simulink model "SC_617_HOMEWORK_2"  (R2025a)
settings: Solver=VariableStepAuto  StartTime=0.0  StopTime=50  RelTol=1e-3
InitFcn:
  | init_params
values from neighbouring files (symbols this model uses):
  A1 = 0.4 * I3    [init_params.m]
  A2 = 0.1 * I3    [init_params.m]
  G = [0; 0; -g]    [init_params.m]
  J = diag([0.00235, 0.00235, 0.0526])    [init_params.m]
  J_inv = inv(J)    [init_params.m]
  K1 = 1 * I3    [init_params.m]
  K2 = 0.01 * I3    [init_params.m]
  X1 = -A1*A1 + I3    [init_params.m]
  X2 = -A2*A2 + I3    [init_params.m]
  Y1 = A1 + Q1 + K1    [init_params.m]
  Y2 = A2 + Q2 + K2    [init_params.m]
libraries: matrix_library x1
settings Model: Creator=bhuvn  LastModifiedBy=bhuvn

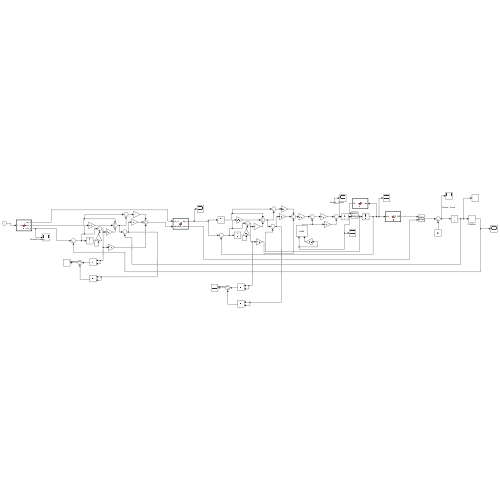
[thumbnail: Simulink's stored preview of the top-level diagram]
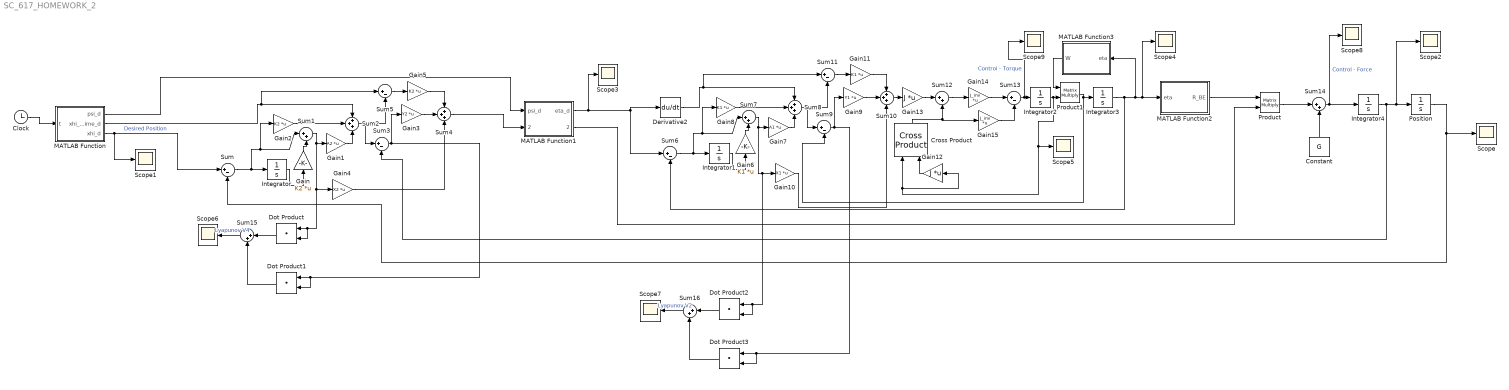
== system SC_617_HOMEWORK_2 ==
  Clock : Clock
  Constant : Constant  Value=G
  Cross Product : matrix_library/Cross Product
  Derivative2 : Derivative
  Dot Product{,1..3} (4 alike) : DotProduct  OutDataTypeStr=Inherit: Inherit via internal rule
  Gain : Gain  Gain=K2  Multiplication=Matrix(K*u)
  Gain1 : Gain  Gain=A2  Multiplication=Matrix(K*u)
  Gain10 : Gain  Gain=X1  Multiplication=Matrix(K*u)
  Gain11 : Gain  Gain=K1  Multiplication=Matrix(K*u)
  Gain12 : Gain  Gain=J  Multiplication=Matrix(K*u)
  Gain13 : Gain  Gain=J  Multiplication=Matrix(K*u)
  Gain14 : Gain  Gain=J_inv  Multiplication=Matrix(K*u)
  Gain15 : Gain  Gain=J_inv  Multiplication=Matrix(K*u)
  Gain2 : Gain  Gain=K2  Multiplication=Matrix(K*u)
  Gain3 : Gain  Gain=Y2  Multiplication=Matrix(K*u)
  Gain4 : Gain  Gain=X2  Multiplication=Matrix(K*u)
  Gain5 : Gain  Gain=K2  Multiplication=Matrix(K*u)
  Gain6 : Gain  Gain=K1  Multiplication=Matrix(K*u)
  Gain7 : Gain  Gain=A1  Multiplication=Matrix(K*u)
  Gain8 : Gain  Gain=K1  Multiplication=Matrix(K*u)
  Gain9 : Gain  Gain=Y1  Multiplication=Matrix(K*u)
  Integrator{,1..4} (5 alike) : Integrator
  MATLAB Function : MATLAB Function  TreatAsAtomicUnit=on
  MATLAB Function1 : MATLAB Function  TreatAsAtomicUnit=on
  MATLAB Function2 : MATLAB Function  TreatAsAtomicUnit=on
  MATLAB Function3 : MATLAB Function  TreatAsAtomicUnit=on
  Position : Integrator  ContinuousStateAttributes="\"\""
  Product : Product  Multiplication=Matrix(*)
  Product1 : Product  Multiplication=Matrix(*)
  Scope{,1..9} (10 alike) : Scope
      Scope settings: ActiveDisplayYMinimum=-4.4635582145538866  ActiveDisplayYMaximum=9.864933478588199
      Scope1 settings: ActiveDisplayYMinimum=-8.7534376610536011  ActiveDisplayYMaximum=9.9256887521870869
      Scope2 settings: ActiveDisplayYMinimum=-1.1742628607223897  ActiveDisplayYMaximum=2.1905461290166537  DataLoggingVariableName=ScopeData2
      Scope3 settings: ActiveDisplayYMinimum=-0.36738889438246891  ActiveDisplayYMaximum=0.46299980810775304  DataLoggingVariableName=ScopeData3
      Scope4 settings: ActiveDisplayYMinimum=-0.8680947606325895  ActiveDisplayYMaximum=0.33111411374778932  DataLoggingVariableName=ScopeData4
      Scope5 settings: ActiveDisplayYMinimum=-5.3845863313289479  ActiveDisplayYMaximum=8.3533958672384383  DataLoggingVariableName=ScopeData5
      Scope6 settings: ActiveDisplayYMinimum=0.017644834477093529  ActiveDisplayYMaximum=1.7083666755814968  DataLoggingVariableName=ScopeData6
      Scope7 settings: ActiveDisplayYMinimum=-0.096269739376810465  ActiveDisplayYMaximum=0.17835060014207538  DataLoggingVariableName=ScopeData7
      Scope8 settings: ActiveDisplayYMinimum=-1.5602667584024623  ActiveDisplayYMaximum=1.6746897222216022  DataLoggingVariableName=ScopeData8
      Scope9 settings: ActiveDisplayYMinimum=-0.8680947606325895  ActiveDisplayYMaximum=0.33111411374778932  DataLoggingVariableName=ScopeData9
  Sum{,3,5..6,9,11,13} (7 alike) : Sum  Inputs=|+-
  Sum{1,7,12,14..16} (6 alike) : Sum  Inputs=|++
  Sum{2,4,8,10} (4 alike) : Sum  Inputs=+++
  wires:
  Clock/1 -> MATLAB Function/1(t)
  MATLAB Function/3(xhi_d) -> Scope1/1, Sum/1  "Desired Position"
  Sum/1 -> Sum1/1, Gain2/1, Integrator/1
  Gain/1 -> Sum1/2
  Integrator/1 -> Gain/1
  MATLAB Function/2(xhi_prime_d) -> Sum5/1, Sum2/1
  Sum1/1 -> Dot Product/2, Dot Product/1, Gain4/1, Gain1/1
  Gain1/1 -> Sum2/3
  Gain2/1 -> Sum2/2
  Sum2/1 -> Sum5/2, Sum3/1
  Sum3/1 -> Gain3/1, Dot Product1/2, Dot Product1/1
  Gain3/1 -> Sum4/2
  Gain4/1 -> Sum4/3
  Sum5/1 -> Gain5/1
  Gain5/1 -> Sum4/1
  MATLAB Function/1(psi_d) -> MATLAB Function1/1(psi_d)
  Gain10/1 -> Sum10/3
  Sum11/1 -> Gain11/1
  Gain11/1 -> Sum10/1
  Integrator1/1 -> Gain6/1
  Gain7/1 -> Sum8/3
  Derivative2/1 -> Sum11/1, Sum8/1
  Gain8/1 -> Sum8/2
  Sum6/1 -> Sum7/1, Gain8/1, Integrator1/1
  Gain9/1 -> Sum10/2
  Sum9/1 -> Dot Product3/2, Dot Product3/1, Gain9/1
  Sum8/1 -> Sum11/2, Sum9/1
  Gain6/1 -> Sum7/2
  Sum7/1 -> Dot Product2/2, Dot Product2/1, Gain10/1, Gain7/1
  Cross Product/1 -> Gain15/1, Sum12/2
  Sum10/1 -> Gain13/1
  Gain13/1 -> Sum12/1
  Sum12/1 -> Gain14/1
  Gain14/1 -> Sum13/1
  Sum13/1 -> Scope9/1, Integrator2/1  "Control - Torque"
  Integrator3/1 -> Sum6/2, MATLAB Function3/1(eta), MATLAB Function2/1(eta), Scope4/1
  MATLAB Function2/1(R_BE) -> Product/1
  Product/1 -> Sum14/1
  Sum14/1 -> Integrator4/1, Scope8/1  "Control - Force"
  Integrator4/1 -> Sum3/2, Scope2/1, Position/1
  Position/1 -> Sum/2, Scope/1
  Integrator2/1 -> Scope5/1, Cross Product/1, Gain12/1, Product1/2
  Product1/1 -> Sum9/2, Integrator3/1
  MATLAB Function3/1(W) -> Product1/1
  MATLAB Function1/1(eta_d) -> Scope3/1, Sum6/1, Derivative2/1
  MATLAB Function1/2(L_vector) -> Product/2
  Gain15/1 -> Sum13/2
  Gain12/1 -> Cross Product/2
  Constant/1 -> Sum14/2
  Sum4/1 -> MATLAB Function1/2(alpha4)
  Dot Product/1 -> Sum15/1
  Dot Product1/1 -> Sum15/2
  Sum15/1 -> Scope6/1  "Lyapunov V4"
  Sum16/1 -> Scope7/1  "Lyapunov V2"
  Dot Product2/1 -> Sum16/1
  Dot Product3/1 -> Sum16/2

== matlab function SC_617_HOMEWORK_2/MATLAB Function1 ==
  data: psi_d input; eta_d output; alpha4 input; L_vector output
function [eta_d, L_vector] = F1(psi_d, alpha4)

    % --- Parameters ---
    g = 9.81;
    m = 2.0; % Mass is needed for Eq. 46
    
    % --- 1. Get Accelerations (U1, U2, U3 from Eq. 44) ---
    ux = alpha4(1);
    uy = alpha4(2);
    uz = alpha4(3); % Vertical acceleration (without g)
    
    % --- 2. Calculate the Norm (Denominator of Eq. 45) ---
    % This represents the total acceleration magnitude
    acc_total_z = uz + g;
    acc_norm = sqrt(ux^2 + uy^2 + acc_total_z^2);
    
    % Safety: Prevent division by zero


    % --- 3. Calculate Thrust Force (Eq. 46) ---
    % The plant needs FORCE (Newtons), so we multiply by mass
    Thrust_Force = acc_norm;
    L_vector = [0; 0; Thrust_Force];

    % --- 4. Calculate Angles (Eq. 45) ---
    % Numerator terms from Eq. 45
    % Note: The paper uses U1, U2 for x, y accel. 
    % We simply rotate them by Yaw (psi_d) as shown in the formula.
    
    % "Lateral" component for Roll (Top part of Eq 45 phi_d)
    num_phi = ux * sin(psi_d) - uy * cos(psi_d);
    
    % "Longitudinal" component for Pitch (Top part of Eq 45 theta_d)
    num_theta = ux * cos(psi_d) + uy * sin(psi_d);
    
    % --- PITCH (Theta) ---
    % Eq 45: theta_d = atan( num_theta / (U3 + g) )
    theta_d = atan(num_theta / acc_total_z);

    % --- ROLL (Phi) ---
    % Eq 45: phi_d = asin( num_phi / acc_norm )
    
    % SAFETY CLAMP: Ensure ratio is between -1 and 1
    phi_arg = num_phi / acc_norm;

    phi_d = asin(phi_arg);

    % --- Pack Outputs ---
    eta_d = [phi_d; theta_d; psi_d];
    
end

== matlab function SC_617_HOMEWORK_2/MATLAB Function ==
  data: psi_d output; xhi_prime_d output; t input; xhi_d output
function [psi_d, xhi_prime_d, xhi_d] = F(t)


    R = 1.0;         % Radius of spiral (m)
    w = 0.5;         % Angular frequency (rad/s)
    z_speed = 0.2;   % Vertical climb speed (m/s)  % Final height (m)

    z = t*z_speed;

    x = R * cos(w * t);
    y = R * sin(w * t);
    x_prime = -R*w*sin(w*t);
    y_prime = R*w*cos(w*t);





    xhi_d = [x; y; z];
    xhi_prime_d = [x_prime; y_prime; z_speed];

    psi_d = 0; 
end

== matlab function SC_617_HOMEWORK_2/MATLAB Function2 ==
  data: eta input; R_BE output
function R_BE = F2(eta)
    % INPUT:
    % eta = [phi; theta; psi] (Roll, Pitch, Yaw in radians)
    
    % OUTPUT:
    % R_EB = 3x3 Rotation Matrix from Inertial (Earth) to Body Frame
    %        (As defined in Eq. 1 of your paper)

    phi   = eta(1);
    theta = eta(2);
    psi   = eta(3);

    % Pre-calculate trig values for readability and speed
    c_phi = cos(phi);   s_phi = sin(phi);
    c_theta = cos(theta); s_theta = sin(theta);
    c_psi = cos(psi);   s_psi = sin(psi);

    % Construct the Matrix (Row by Row)
    % Row 1
    r11 = c_psi * c_theta;
    r12 = c_theta * s_psi;
    r13 = -s_theta;

    % Row 2
    r21 = c_psi * s_phi * s_theta - c_phi * s_psi;
    r22 = c_phi * c_psi + s_phi * s_psi * s_theta;
    r23 = c_theta * s_phi;

    % Row 3
    r31 = s_phi * s_psi + c_phi * c_psi * s_theta;
    r32 = c_phi * s_psi * s_theta - c_psi * s_phi;
    r33 = c_phi * c_theta;

    % Combine into matrix
    R_BE = [r11, r21, r31;
            r12, r22, r32;
            r13, r23, r33];
end

== matlab function SC_617_HOMEWORK_2/MATLAB Function3 ==
  data: eta input; W output size=[3 3]
function W = F3(eta)


    phi   = eta(1);
    theta = eta(2);

    s_phi = sin(phi);
    c_phi = cos(phi);
    t_theta = tan(theta);
    
    c_theta = cos(theta);

    sec_theta = 1 / c_theta;


    w11 = 1;
    w12 = s_phi * t_theta;
    w13 = c_phi * t_theta;


    w21 = 0;
    w22 = c_phi;
    w23 = -s_phi;


    w31 = 0;
    w32 = s_phi * sec_theta; % Equivalent to sin(phi)/cos(theta)
    w33 = c_phi * sec_theta; % Equivalent to cos(phi)/cos(theta)

    W = [w11, w12, w13;
         w21, w22, w23;
         w31, w32, w33];
end
